simulink model "PubIfDecisionLM_MDL"  (R2020b)
settings: configuration reference "DspaceConfig" (kept outside this file)
PostLoadFcn:
  | if any(exist('dsrtsu_mdlpostloadfcn', 'file') ~= 0), dsrtsu_mdlpostloadfcn('Execute', bdroot); end
InitFcn:
  | , if any(exist('dsmpb_private', 'file') ~= 0), dsmpb_private('dsmpb_mdlclblib', 'Init', bdroot); end,
undefined symbols (not defined in the file or in its folder): OFM_OBJ_FUSIONTYPE_E, OFM_OBJ_MOVINGSTATE_E, OFM_OBJ_ORIENTATION_E, OFM_OBJ_TYPE_E, P_LM_Cyc, P_LM_EMLHistKapRcdBufSize, P_LM_EMLHistTrajBaseDis, P_LM_EMLHistTrajPNum, P_LM_EMLKapCorrMaxThre, P_LM_EMLMinKapThre, P_LM_EMLPathDisDiffThre, P_LM_EMLQuaFiltPar, P_LM_EMLTurnActKapThre, P_LM_EMLValidQuaThre, P_LM_FntPath1Disgap, P_LM_FntPath1MinDis, P_LM_FntPath1Timegap, P_LM_FntPath2Disgap, P_LM_FntPath2MinDis, P_LM_FntPath2Timegap, P_LM_FntPath3Disgap, P_LM_FntPath3MinDis, P_LM_FntPath3Timegap, P_LM_FusBLParFiltP, P_LM_FusEVDifC2Thre, P_LM_FusEVOPath1AllVSLDisThre, P_LM_FusEVOPath1AllVSLLostNumThre, P_LM_FusEVOPath1AllVSLQuaThre, P_LM_FusEVOPath1OTLFacNLC, P_LM_FusOTLQuaThre, P_LM_FusOTLSW, P_LM_FusParC0Index, P_LM_FusParC1Index, P_LM_FusParC2Index, P_LM_FusParC3Index, P_LM_FusVSLQuaThre, P_LM_FusVSLSW, P_LM_FusVSLValidSteerWheerAngThre, P_LM_FusVSLValidVxvThre, P_LM_LaneWidth, P_LM_OTLBufTPInfoEvaFactor, P_LM_OTLObjNum, P_LM_OTLObjSelectAgeThre, P_LM_OTLObjSelectDxAssessVx, P_LM_OTLObjSelectDxThre, P_LM_OTLObjSelectVxThre, P_LM_OTLObjSelectVyAssessDx, P_LM_OTLObjSelectVyThre, P_LM_OTLTrajPntBaseDis, P_LM_OTLTrajStdThre, P_LM_VSLAvailLineNum, P_LM_VSLBLSDiffThre, P_LM_VSLBLSDisRatio, P_LM_VSLFusBLParFiltP_C1, P_LM_VSLFusBLParFiltP_C2, P_LM_VSLFusBLParFiltP_C3, P_LM_VSLFusBLParFiltP_Quality, P_LM_VSLHistTrajBaseDis, P_LM_VSLHistTrajPNum, P_LM_VSLLCC0diff ... (+18)
libraries: simulink x145, LM_LIB x43
(part 12 of 24)

== system PubIfDecisionLM_MDL/Subsystem2/LM_Fusion1/LM_FusRatioCalc/LM_Fusion_EVO/LM_FusEVORatioCalc/LM_Fusion_FntPathK ==
  LM_EMLFntPath1Quality : Inport
  LM_EMLFntPath2Quality : Inport  Port=2
  LM_EMLFntPath3Quality : Inport  Port=3
  LM_VSLFntPath1Quality : Inport  Port=4
  LM_VSLFntPath2Quality : Inport  Port=5
  LM_VSLFntPath3Quality : Inport  Port=6
  LM_VSLBaseDis : Inport  Port=7
  LM_OTLFntPath1Qulity : Inport  Port=8
  LM_OTLFntPath2Qulity : Inport  Port=9
  LM_OTLFntPath3Qulity : Inport  Port=10
  LM_ComLineLostNum : Inport  Port=11
  LM_FntPath1Dis : Inport  Port=12
  LM_FntPath2Dis : Inport  Port=13
  vxvRefMs : Inport  Port=14
  DIR_TurnLeftValid : Inport  Port=15
  DIR_TurnRightValid : Inport  Port=16
  DIR_LC2LeValid : Inport  Port=17
  DIR_LC2RigValid : Inport  Port=18
  LM_FusEVOFntPath1 : Subsystem
  LM_FusEVOFntPath2 : Subsystem
  LM_FusEVOFntPath3 : Subsystem
  LM_FusEVOFntPath1EMLK : Outport
  LM_FusEVOFntPath1VSLK : Outport  Port=2
  LM_FusEVOFntPath1OTLK : Outport  Port=3
  LM_FusEVOFntPath1RELK : Outport  Port=4
  LM_FusEVOFntPath1MALK : Outport  Port=5
  LM_FusEVOFntPath2EMLK : Outport  Port=6
  LM_FusEVOFntPath2VSLK : Outport  Port=7
  LM_FusEVOFntPath2OTLK : Outport  Port=8
  LM_FusEVOFntPath2RELK : Outport  Port=9
  LM_FusEVOFntPath2MALK : Outport  Port=10
  LM_FusEVOFntPath3EMLK : Outport  Port=11
  LM_FusEVOFntPath3VSLK : Outport  Port=12
  LM_FusEVOFntPath3OTLK : Outport  Port=13
  LM_FusEVOFntPath3RELK : Outport  Port=14
  LM_FusEVOFntPath3MALK : Outport  Port=15
  wires:
  LM_EMLFntPath1Quality/1 -> LM_FusEVOFntPath1/1(LM_EMLFntPath1Quality)
  LM_VSLFntPath1Quality/1 -> LM_FusEVOFntPath1/2(LM_VSLFntPath1Quality)
  LM_VSLBaseDis/1 -> LM_FusEVOFntPath2/7(LM_VSLBaseDis), LM_FusEVOFntPath1/3(LM_VSLBaseDis)
  LM_OTLFntPath1Qulity/1 -> LM_FusEVOFntPath1/4(LM_OTLFntPath1Qulity)
  LM_ComLineLostNum/1 -> LM_FusEVOFntPath3/1(LM_ComLineLostNum), LM_FusEVOFntPath2/1(LM_ComLineLostNum), LM_FusEVOFntPath1/5(LM_ComLineLostNum)
  LM_FntPath1Dis/1 -> LM_FusEVOFntPath1/6(LM_FntPath1Dis)
  vxvRefMs/1 -> LM_FusEVOFntPath3/7(vxvRefMs), LM_FusEVOFntPath2/9(vxvRefMs), LM_FusEVOFntPath1/7(vxvRefMs)
  LM_EMLFntPath2Quality/1 -> LM_FusEVOFntPath2/2(LM_EMLFntPath2Quality)
  LM_VSLFntPath2Quality/1 -> LM_FusEVOFntPath2/3(LM_VSLFntPath2Quality)
  LM_OTLFntPath2Qulity/1 -> LM_FusEVOFntPath2/4(LM_OTLFntPath2Qulity)
  LM_FusEVOFntPath1/1(LM_FusEVOFntPath1EMLK) -> LM_FusEVOFntPath1EMLK/1
  LM_FusEVOFntPath1/2(LM_FusEVOFntPath1VSLK) -> LM_FusEVOFntPath1VSLK/1
  LM_FusEVOFntPath1/3(LM_FusEVOFntPath1OTLK) -> LM_FusEVOFntPath1OTLK/1
  LM_FusEVOFntPath2/1(LM_FusEVOFntPath2EMLK) -> LM_FusEVOFntPath2EMLK/1
  LM_FusEVOFntPath2/2(LM_FusEVOFntPath2VSLK) -> LM_FusEVOFntPath2VSLK/1
  LM_FusEVOFntPath2/3(LM_FusEVOFntPath2OTLK) -> LM_FusEVOFntPath2OTLK/1
  LM_FusEVOFntPath1/4(LM_FusEVOFntPath1RELK) -> LM_FusEVOFntPath1RELK/1
  LM_FusEVOFntPath1/5(LM_FusEVOFntPath1MALK) -> LM_FusEVOFntPath1MALK/1
  LM_FusEVOFntPath2/4(LM_FusEVOFntPath2RELK) -> LM_FusEVOFntPath2RELK/1
  LM_FusEVOFntPath2/5(LM_FusEVOFntPath2MALK) -> LM_FusEVOFntPath2MALK/1
  LM_OTLFntPath3Qulity/1 -> LM_FusEVOFntPath3/4(LM_OTLFntPath3Quality)
  LM_VSLFntPath3Quality/1 -> LM_FusEVOFntPath3/3(LM_VSLFntPath3Quality)
  LM_EMLFntPath3Quality/1 -> LM_FusEVOFntPath3/2(LM_EMLFntPath3Quality)
  LM_FusEVOFntPath3/1(LM_FusEVOFntPath3EMLK) -> LM_FusEVOFntPath3EMLK/1
  LM_FusEVOFntPath3/2(LM_FusEVOFntPath3VSLK) -> LM_FusEVOFntPath3VSLK/1
  LM_FusEVOFntPath3/3(LM_FusEVOFntPath3OTLK) -> LM_FusEVOFntPath3OTLK/1
  LM_FusEVOFntPath3/4(LM_FusEVOFntPath3RELK) -> LM_FusEVOFntPath3RELK/1
  LM_FusEVOFntPath3/5(LM_FusEVOFntPath3MALK) -> LM_FusEVOFntPath3MALK/1
  DIR_TurnLeftValid/1 -> LM_FusEVOFntPath2/5(DIR_TurnLeftValid), LM_FusEVOFntPath3/5(DIR_TurnLeftValid), LM_FusEVOFntPath1/8(DIR_TurnLeftValid)
  DIR_TurnRightValid/1 -> LM_FusEVOFntPath3/6(DIR_TurnRightValid), LM_FusEVOFntPath2/6(DIR_TurnRightValid), LM_FusEVOFntPath1/9(DIR_TurnRightValid)
  DIR_LC2LeValid/1 -> LM_FusEVOFntPath1/10(DIR_LC2LeValid), LM_FusEVOFntPath2/10(DIR_LC2LeValid), LM_FusEVOFntPath3/8(DIR_LC2LeValid)
  DIR_LC2RigValid/1 -> LM_FusEVOFntPath1/11(DIR_LC2RigValid), LM_FusEVOFntPath2/11(DIR_LC2RigValid), LM_FusEVOFntPath3/9(DIR_LC2RigValid)
  LM_FntPath2Dis/1 -> LM_FusEVOFntPath2/8(LM_FntPath2Dis)

== system PubIfDecisionLM_MDL/Subsystem2/LM_Fusion1/LM_FusRatioCalc/LM_Fusion_EVO/LM_FusEVORatioCalc/LM_Fusion_RearPathK ==
  Constant{,1..5} (6 alike) : Constant  Value=0  OutDataTypeStr=single
  LM_FusRearPath1VSLK : Outport
  LM_FusRearPath2VSLK : Outport  Port=2
  LM_FusRearPath3VSLK : Outport  Port=3
  LM_FusRearPath1EMLK : Outport  Port=4
  LM_FusRearPath2EMLK : Outport  Port=5
  LM_FusRearPath3EMLK : Outport  Port=6
  wires:
  Constant3/1 -> LM_FusRearPath2EMLK/1  "LM_FusRearPath2EMLK"
  Constant4/1 -> LM_FusRearPath3VSLK/1  "LM_FusRearPath3VSLK"
  Constant5/1 -> LM_FusRearPath3EMLK/1  "LM_FusRearPath3EMLK"
  Constant2/1 -> LM_FusRearPath2VSLK/1  "LM_FusRearPath2VSLK"
  Constant1/1 -> LM_FusRearPath1EMLK/1  "LM_FusRearPath1EMLK"
  Constant/1 -> LM_FusRearPath1VSLK/1  "LM_FusRearPath1VSLK"

== system PubIfDecisionLM_MDL/Subsystem2/LM_Fusion1/LM_Fus_BLConnectivityCheck/LM_Fus_BLFntPahtConnectivityCheck/LM_Fus_BLFntPahtConnectivityCheck/LM_Fus_BLFntPath1Info ==
  LM_FusBLFntPath1Quality : Inport
  LM_FusBLFntPath1C0 : Inport  Port=2
  LM_FusBLFntPath1C1 : Inport  Port=3
  LM_FusBLFntPath1C2 : Inport  Port=4
  LM_FusBLFntPath1C3 : Inport  Port=5
  Signal Conversion{,1..4} (5 alike) : SignalConversion  OverrideOpt=off
  LM_FusBLFntPath1C0Adju : Outport
  LM_FusBLFntPath1C1Adju : Outport  Port=2
  LM_FusBLFntPath1C2Adju : Outport  Port=3
  LM_FusBLFntPath1C3Adju : Outport  Port=4
  LM_FusBLFntPath1QualityAdju : Outport  Port=5
  wires:
  LM_FusBLFntPath1C2/1 -> Signal Conversion2/1
  LM_FusBLFntPath1C0/1 -> Signal Conversion/1
  LM_FusBLFntPath1C1/1 -> Signal Conversion1/1
  LM_FusBLFntPath1Quality/1 -> Signal Conversion4/1
  LM_FusBLFntPath1C3/1 -> Signal Conversion3/1
  Signal Conversion/1 -> LM_FusBLFntPath1C0Adju/1  "LM_FusBLFntPath1C0Adju"
  Signal Conversion1/1 -> LM_FusBLFntPath1C1Adju/1  "LM_FusBLFntPath1C1Adju"
  Signal Conversion2/1 -> LM_FusBLFntPath1C2Adju/1  "LM_FusBLFntPath1C2Adju"
  Signal Conversion3/1 -> LM_FusBLFntPath1C3Adju/1  "LM_FusBLFntPath1C3Adju"
  Signal Conversion4/1 -> LM_FusBLFntPath1QualityAdju/1  "LM_FusBLFntPath1QualityAdju"

== system PubIfDecisionLM_MDL/Subsystem2/LM_Fusion1/LM_Fus_BLConnectivityCheck/LM_Fus_BLFntPahtConnectivityCheck/LM_Fus_BLFntPahtConnectivityCheck/LM_Fus_BLFntPath2Info ==
  LM_FusBLFntPath1C0 : Inport
  LM_FusBLFntPath1C1 : Inport  Port=2
  LM_FusBLFntPath1C2 : Inport  Port=3
  LM_FusBLFntPath1C3 : Inport  Port=4
  LM_FusBLFntPath2Quality : Inport  Port=5
  LM_FusBLFntPath2C0BefAduj : Inport  Port=6
  LM_FusBLFntPath2C1 : Inport  Port=7
  LM_FusBLFntPath2C2 : Inport  Port=8
  LM_FusBLFntPath2C3 : Inport  Port=9
  LM_FntPath1Dis : Inport  Port=10
  LM_Fus_BLFntPath2C0Adju : Subsystem
  LM_Fus_BLFntPath2Info : Subsystem
  LM_FusBLFntPath2C0Adju : Outport
  LM_FusBLFntPath2C1Adju : Outport  Port=2
  LM_FusBLFntPath2C2Adju : Outport  Port=3
  LM_FusBLFntPath2C3Adju : Outport  Port=4
  LM_FusBLFntPath2QualityAdju : Outport  Port=5
  wires:
  LM_FusBLFntPath1C0/1 -> LM_Fus_BLFntPath2C0Adju/1(LM_FusBLFntPath1C0)
  LM_FusBLFntPath1C1/1 -> LM_Fus_BLFntPath2C0Adju/2(LM_FusBLFntPath1C1)
  LM_FusBLFntPath1C2/1 -> LM_Fus_BLFntPath2C0Adju/3(LM_FusBLFntPath1C2)
  LM_FusBLFntPath1C3/1 -> LM_Fus_BLFntPath2C0Adju/4(LM_FusBLFntPath1C3)
  LM_FntPath1Dis/1 -> LM_Fus_BLFntPath2C0Adju/5(LM_FntPath1Dis)
  LM_FusBLFntPath2C0BefAduj/1 -> LM_Fus_BLFntPath2C0Adju/6(LM_FusBLFntPath2C0BefAduj)
  LM_FusBLFntPath2C1/1 -> LM_Fus_BLFntPath2C0Adju/7(LM_FusBLFntPath2C1), LM_Fus_BLFntPath2Info/2(LM_FusBLFntPath2C1)
  LM_FusBLFntPath2C2/1 -> LM_Fus_BLFntPath2C0Adju/8(LM_FusBLFntPath2C2), LM_Fus_BLFntPath2Info/3(LM_FusBLFntPath2C2)
  LM_FusBLFntPath2C3/1 -> LM_Fus_BLFntPath2C0Adju/9(LM_FusBLFntPath2C3), LM_Fus_BLFntPath2Info/4(LM_FusBLFntPath2C3)
  LM_Fus_BLFntPath2C0Adju/1(LM_FusBLFntPath2C0Aduj) -> LM_Fus_BLFntPath2Info/1(LM_FusBLFntPath2C0Aduj)
  LM_FusBLFntPath2Quality/1 -> LM_Fus_BLFntPath2Info/5(LM_FusBLFntPath2Quality)
  LM_Fus_BLFntPath2Info/5(LM_FusBLFntPath2QualityAdju) -> LM_FusBLFntPath2QualityAdju/1
  LM_Fus_BLFntPath2Info/4(LM_FusBLFntPath2C3Adju) -> LM_FusBLFntPath2C3Adju/1
  LM_Fus_BLFntPath2Info/2(LM_FusBLFntPath2C1Adju) -> LM_FusBLFntPath2C1Adju/1
  LM_Fus_BLFntPath2Info/3(LM_FusBLFntPath2C2Adju) -> LM_FusBLFntPath2C2Adju/1
  LM_Fus_BLFntPath2Info/1(LM_FusBLFntPath2C0Adju) -> LM_FusBLFntPath2C0Adju/1

== system PubIfDecisionLM_MDL/Subsystem2/LM_Fusion1/LM_Fus_BLConnectivityCheck/LM_Fus_BLFntPahtConnectivityCheck/LM_Fus_BLFntPahtConnectivityCheck/LM_Fus_BLFntPath3Info ==
  LM_FusBLFntPath2C0Aduj : Inport
  LM_FusBLFntPath2C1 : Inport  Port=2
  LM_FusBLFntPath2C2 : Inport  Port=3
  LM_FusBLFntPath2C3 : Inport  Port=4
  LM_FusBLFntPath3C0BefAduj : Inport  Port=5
  LM_FusBLFntPath3C1 : Inport  Port=6
  LM_FusBLFntPath3C2 : Inport  Port=7
  LM_FusBLFntPath3C3 : Inport  Port=8
  LM_FusBLFntPath3Quality : Inport  Port=9
  LM_FntPath2Dis : Inport  Port=10
  LM_Fus_BLFntPath2C0Adju : Subsystem
  LM_Fus_BLFntPath2Info : Subsystem
  LM_FusBLFntPath3C0Adju : Outport
  LM_FusBLFntPath3C1Adju : Outport  Port=2
  LM_FusBLFntPath3C2Adju : Outport  Port=3
  LM_FusBLFntPath3C3Adju : Outport  Port=4
  LM_FusBLFntPath3QualityAdju : Outport  Port=5
  wires:
  LM_Fus_BLFntPath2C0Adju/1(LM_FusBLFntPath3C0Aduj) -> LM_Fus_BLFntPath2Info/1(LM_FusBLFntPath3C0Aduj)
  LM_FusBLFntPath3Quality/1 -> LM_Fus_BLFntPath2Info/5(LM_FusBLFntPath3Quality)
  LM_FusBLFntPath3C1/1 -> LM_Fus_BLFntPath2Info/2(LM_FusBLFntPath3C1), LM_Fus_BLFntPath2C0Adju/7(LM_FusBLFntPath3C1)
  LM_FusBLFntPath3C2/1 -> LM_Fus_BLFntPath2Info/3(LM_FusBLFntPath3C2), LM_Fus_BLFntPath2C0Adju/8(LM_FusBLFntPath3C2)
  LM_FusBLFntPath3C3/1 -> LM_Fus_BLFntPath2Info/4(LM_FusBLFntPath3C3), LM_Fus_BLFntPath2C0Adju/9(LM_FusBLFntPath3C3)
  LM_FusBLFntPath2C0Aduj/1 -> LM_Fus_BLFntPath2C0Adju/1(LM_FusBLFntPath2C0)
  LM_FusBLFntPath2C1/1 -> LM_Fus_BLFntPath2C0Adju/2(LM_FusBLFntPath2C1)
  LM_FusBLFntPath2C2/1 -> LM_Fus_BLFntPath2C0Adju/3(LM_FusBLFntPath2C2)
  LM_FusBLFntPath2C3/1 -> LM_Fus_BLFntPath2C0Adju/4(LM_FusBLFntPath2C3)
  LM_FntPath2Dis/1 -> LM_Fus_BLFntPath2C0Adju/5(LM_FntPath2Dis)
  LM_FusBLFntPath3C0BefAduj/1 -> LM_Fus_BLFntPath2C0Adju/6(LM_FusBLFntPath3C0BefAduj)
  LM_Fus_BLFntPath2Info/3(LM_FusBLFntPath3C2Adju) -> LM_FusBLFntPath3C2Adju/1
  LM_Fus_BLFntPath2Info/2(LM_FusBLFntPath3C1Adju) -> LM_FusBLFntPath3C1Adju/1
  LM_Fus_BLFntPath2Info/4(LM_FusBLFntPath3C3Adju) -> LM_FusBLFntPath3C3Adju/1
  LM_Fus_BLFntPath2Info/1(LM_FusBLFntPath3C0Adju) -> LM_FusBLFntPath3C0Adju/1
  LM_Fus_BLFntPath2Info/5(LM_FusBLFntPath3QualityAdju) -> LM_FusBLFntPath3QualityAdju/1

== system PubIfDecisionLM_MDL/Subsystem2/LM_Fusion1/LM_Fus_BLConnectivityCheck/LM_Fus_BLRearPahtConnectivityCheck/LM_Fus_BLRearPahtConnectivityCheck/LM_Fus_BLFntPath2Info ==
  LM_FusBLRearPath1C0 : Inport
  LM_FusBLRearPath1C1 : Inport  Port=2
  LM_FusBLRearPath1C2 : Inport  Port=3
  LM_FusBLRearPath1C3 : Inport  Port=4
  LM_FusBLRearPath2Quality : Inport  Port=5
  LM_FusBLFntPath2C0BefAduj : Inport  Port=6
  LM_FusBLRearPath2C1 : Inport  Port=7
  LM_FusBLRearPath2C2 : Inport  Port=8
  LM_FusBLRearPath2C3 : Inport  Port=9
  LM_RearPath1Dis : Inport  Port=10
  LM_Fus_BLFntPath2C0Adju : Subsystem
  LM_Fus_BLFntPath2Info : Subsystem
  LM_FusBLRearPath2C0Adju : Outport
  LM_FusBLRearPath2C1Adju : Outport  Port=2
  LM_FusBLRearPath2C2Adju : Outport  Port=3
  LM_FusBLRearPath2C3Adju : Outport  Port=4
  LM_FusBLRearPath2QualityAdju : Outport  Port=5
  wires:
  LM_FusBLRearPath1C0/1 -> LM_Fus_BLFntPath2C0Adju/1(LM_FusBLFntPath1C0)
  LM_FusBLRearPath1C1/1 -> LM_Fus_BLFntPath2C0Adju/2(LM_FusBLFntPath1C1)
  LM_FusBLRearPath1C2/1 -> LM_Fus_BLFntPath2C0Adju/3(LM_FusBLFntPath1C2)
  LM_FusBLRearPath1C3/1 -> LM_Fus_BLFntPath2C0Adju/4(LM_FusBLFntPath1C3)
  LM_RearPath1Dis/1 -> LM_Fus_BLFntPath2C0Adju/5(LM_FntPath1Dis)
  LM_FusBLFntPath2C0BefAduj/1 -> LM_Fus_BLFntPath2C0Adju/6(LM_FusBLFntPath2C0BefAduj)
  LM_FusBLRearPath2C1/1 -> LM_Fus_BLFntPath2C0Adju/7(LM_FusBLFntPath2C1), LM_Fus_BLFntPath2Info/2(LM_FusBLFntPath2C1)
  LM_FusBLRearPath2C2/1 -> LM_Fus_BLFntPath2C0Adju/8(LM_FusBLFntPath2C2), LM_Fus_BLFntPath2Info/3(LM_FusBLFntPath2C2)
  LM_FusBLRearPath2C3/1 -> LM_Fus_BLFntPath2C0Adju/9(LM_FusBLFntPath2C3), LM_Fus_BLFntPath2Info/4(LM_FusBLFntPath2C3)
  LM_Fus_BLFntPath2C0Adju/1(LM_FusBLFntPath2C0Aduj) -> LM_Fus_BLFntPath2Info/1(LM_FusBLFntPath2C0Aduj)
  LM_FusBLRearPath2Quality/1 -> LM_Fus_BLFntPath2Info/5(LM_FusBLFntPath2Quality)
  LM_Fus_BLFntPath2Info/5(LM_FusBLRearPath2QualityAdju) -> LM_FusBLRearPath2QualityAdju/1
  LM_Fus_BLFntPath2Info/4(LM_FusBLRearPath2C3Adju) -> LM_FusBLRearPath2C3Adju/1
  LM_Fus_BLFntPath2Info/2(LM_FusBLRearPath2C1Adju) -> LM_FusBLRearPath2C1Adju/1
  LM_Fus_BLFntPath2Info/3(LM_FusBLRearPath2C2Adju) -> LM_FusBLRearPath2C2Adju/1
  LM_Fus_BLFntPath2Info/1(LM_FusBLRearPath2C0Adju) -> LM_FusBLRearPath2C0Adju/1

== system PubIfDecisionLM_MDL/Subsystem2/LM_Fusion1/LM_Fus_BLConnectivityCheck/LM_Fus_BLRearPahtConnectivityCheck/LM_Fus_BLRearPahtConnectivityCheck/LM_Fus_BLFntPath3Info ==
  LM_FusBLFntPath2C0Aduj : Inport
  LM_FusBLFntPath2C1 : Inport  Port=2
  LM_FusBLFntPath2C2 : Inport  Port=3
  LM_FusBLFntPath2C3 : Inport  Port=4
  LM_FusBLFntPath3C0BefAduj : Inport  Port=5
  LM_FusBLFntPath3C1 : Inport  Port=6
  LM_FusBLFntPath3C2 : Inport  Port=7
  LM_FusBLFntPath3C3 : Inport  Port=8
  LM_FusBLFntPath3Quality : Inport  Port=9
  LM_FntPath2Dis : Inport  Port=10
  LM_Fus_BLFntPath2Info : Subsystem
  LM_Fus_BLRearPath3C0Adju : Subsystem
  LM_FusBLRearPath3C0Adju : Outport
  LM_FusBLRearPath3C1Adju : Outport  Port=2
  LM_FusBLRearPath3C2Adju : Outport  Port=3
  LM_FusBLRearPath3C3Adju : Outport  Port=4
  LM_FusBLRearPath3QualityAdju : Outport  Port=5
  wires:
  LM_Fus_BLRearPath3C0Adju/1(LM_FusBLFntPath3C0Check) -> LM_Fus_BLFntPath2Info/1(LM_FusBLFntPath3C0Check)
  LM_FusBLFntPath3Quality/1 -> LM_Fus_BLFntPath2Info/5(LM_FusBLFntPath3Quality)
  LM_FusBLFntPath3C1/1 -> LM_Fus_BLFntPath2Info/2(LM_FusBLFntPath3C1), LM_Fus_BLRearPath3C0Adju/7(LM_FusBLFntPath3C1)
  LM_FusBLFntPath3C2/1 -> LM_Fus_BLFntPath2Info/3(LM_FusBLFntPath3C2), LM_Fus_BLRearPath3C0Adju/8(LM_FusBLFntPath3C2)
  LM_FusBLFntPath3C3/1 -> LM_Fus_BLFntPath2Info/4(LM_FusBLFntPath3C3), LM_Fus_BLRearPath3C0Adju/9(LM_FusBLFntPath3C3)
  LM_FusBLFntPath2C0Aduj/1 -> LM_Fus_BLRearPath3C0Adju/1(LM_FusBLFntPath2C0)
  LM_FusBLFntPath2C1/1 -> LM_Fus_BLRearPath3C0Adju/2(LM_FusBLFntPath2C1)
  LM_FusBLFntPath2C2/1 -> LM_Fus_BLRearPath3C0Adju/3(LM_FusBLFntPath2C2)
  LM_FusBLFntPath2C3/1 -> LM_Fus_BLRearPath3C0Adju/4(LM_FusBLFntPath2C3)
  LM_FntPath2Dis/1 -> LM_Fus_BLRearPath3C0Adju/5(LM_FntPath2Dis)
  LM_FusBLFntPath3C0BefAduj/1 -> LM_Fus_BLRearPath3C0Adju/6(LM_FusBLFntPath3C0BefAduj)
  LM_Fus_BLFntPath2Info/2(LM_FusBLRearPath3C1Adju) -> LM_FusBLRearPath3C1Adju/1
  LM_Fus_BLFntPath2Info/3(LM_FusBLRearPath3C2Adju) -> LM_FusBLRearPath3C2Adju/1
  LM_Fus_BLFntPath2Info/1(LM_FusBLRearPath3C0Adju) -> LM_FusBLRearPath3C0Adju/1
  LM_Fus_BLFntPath2Info/4(LM_FusBLRearPath3C3Adju) -> LM_FusBLRearPath3C3Adju/1
  LM_Fus_BLFntPath2Info/5(LM_FusBLRearPath3QualityAdju) -> LM_FusBLRearPath3QualityAdju/1

== system PubIfDecisionLM_MDL/Subsystem2/LM_Fusion1/LM_Fus_BLConnectivityCheck/LM_Fus_BLRearPahtConnectivityCheck/LM_Fus_BLRearPahtConnectivityCheck/LM_Fus_BLRearPath1Info ==
  LM_FusBLFntPath1Quality : Inport
  LM_FusBLFntPath1C0 : Inport  Port=2
  LM_FusBLFntPath1C1 : Inport  Port=3
  LM_FusBLFntPath1C2 : Inport  Port=4
  LM_FusBLFntPath1C3 : Inport  Port=5
  Signal Conversion{,1..4} (5 alike) : SignalConversion  OverrideOpt=off
  LM_FusBLRearPath1C0Adju : Outport
  LM_FusBLRearPath1C1Adju : Outport  Port=2
  LM_FusBLRearPath1C2Adju : Outport  Port=3
  LM_FusBLRearPath1C3Adju : Outport  Port=4
  LM_FusBLRearPath1QualityAdju : Outport  Port=5
  wires:
  Signal Conversion/1 -> LM_FusBLRearPath1C0Adju/1  "LM_FusBLRearPath1C0Adju"
  Signal Conversion2/1 -> LM_FusBLRearPath1C2Adju/1  "LM_FusBLRearPath1C2Adju"
  Signal Conversion4/1 -> LM_FusBLRearPath1QualityAdju/1  "LM_FusBLRearPath1QualityAdju"
  Signal Conversion3/1 -> LM_FusBLRearPath1C3Adju/1  "LM_FusBLRearPath1C3Adju"
  Signal Conversion1/1 -> LM_FusBLRearPath1C1Adju/1  "LM_FusBLRearPath1C1Adju"
  LM_FusBLFntPath1C0/1 -> Signal Conversion/1
  LM_FusBLFntPath1C1/1 -> Signal Conversion1/1
  LM_FusBLFntPath1C2/1 -> Signal Conversion2/1
  LM_FusBLFntPath1C3/1 -> Signal Conversion3/1
  LM_FusBLFntPath1Quality/1 -> Signal Conversion4/1

== system PubIfDecisionLM_MDL/Subsystem2/LM_OTL/LM_OTL_MovObjTrajFit/LM_OTL_BufTPAssess/LM_OTL_BufTrajEva/Subsystem ==
  LM_OTLBufValid : Inport
  LM_OTLBufTPVectBus : Inport  Port=2
  ILM_OTLBufTPInfoBus : Inport  Port=3
  LM_PathDisBus : Inport  Port=4
  Bus Selector : BusSelector  OutputSignals=LM_OTLBufE1Valid
  Bus Selector1 : BusSelector  OutputSignals=LM_OTLBufE1DxVect,LM_OTLBufE1DyVect
  Bus Selector2 : BusSelector  OutputSignals=LM_OTLBufSPPosInfo.LM_OTLBufE1SPPos,LM_OTLBufEPPosInfo.LM_OTLBufE1EPPos
  Bus Selector3 : BusSelector  OutputSignals=LM_PathDisBus.LM_FntPath1Dis,LM_PathDisBus.LM_FntPath2Dis,LM_PathDisBus.LM_FntPath3Dis
  Constant : Constant  Value=P_LM_OTLTrajStdThre
  MATLAB Function1 : MATLAB Function  TreatAsAtomicUnit=on
  LM_OTLBufE1Offset : Outport
  LM_OTLBufE1Flg : Outport  Port=2
  LM_OTLBufE1TpValidNum : Outport  Port=3
  LM_OTLBufE1SPValidPos : Outport  Port=4
  wires:
  Constant/1 -> MATLAB Function1/9(P_LM_OTLTrajStdThre)
  Bus Selector1/1 -> MATLAB Function1/2(LM_OTLDxVect)  "<LM_OTLBufE1DxVect>"
  Bus Selector/1 -> MATLAB Function1/1(LM_OTLBufValidInfo)  "<LM_OTLBufE1Valid>"
  MATLAB Function1/2(Flg) -> LM_OTLBufE1Flg/1
  Bus Selector3/3 -> MATLAB Function1/8(LM_FntPath3Dis)  "<LM_FntPath3Dis>"
  Bus Selector2/1 -> MATLAB Function1/4(LM_OTLSPPos)  "<LM_OTLBufE1SPPos>"
  Bus Selector2/2 -> MATLAB Function1/5(LM_OTLEPPos)  "<LM_OTLBufE1EPPos>"
  Bus Selector1/2 -> MATLAB Function1/3(LM_OTLDyVect)  "<LM_OTLBufE1DyVect>"
  LM_OTLBufValid/1 -> Bus Selector/1
  Bus Selector3/2 -> MATLAB Function1/7(LM_FntPath2Dis)  "<LM_FntPath2Dis>"
  Bus Selector3/1 -> MATLAB Function1/6(LM_FntPath1Dis)  "<LM_FntPath1Dis>"
  MATLAB Function1/1(Offset) -> LM_OTLBufE1Offset/1
  ILM_OTLBufTPInfoBus/1 -> Bus Selector2/1
  LM_OTLBufTPVectBus/1 -> Bus Selector1/1
  LM_PathDisBus/1 -> Bus Selector3/1
  MATLAB Function1/3(TpValidNum) -> LM_OTLBufE1TpValidNum/1
  MATLAB Function1/4(SPValidPos) -> LM_OTLBufE1SPValidPos/1

== system PubIfDecisionLM_MDL/Subsystem2/LM_OTL/LM_OTL_MovObjTrajFit/LM_OTL_BufTPAssess/LM_OTL_BufTrajEva/Subsystem1 ==
  LM_OTLBufValid : Inport
  LM_OTLBufTPVectBus : Inport  Port=2
  ILM_OTLBufTPInfoBus : Inport  Port=3
  LM_PathDisBus : Inport  Port=4
  Bus Selector : BusSelector  OutputSignals=LM_OTLBufL1LastValid
  Bus Selector1 : BusSelector  OutputSignals=LM_OTLBufL1DxVect,LM_OTLBufL1DyVect
  Bus Selector2 : BusSelector  OutputSignals=LM_OTLBufLastSPPosInfo.LM_OTLBufL1LastSPPos,LM_OTLBufLastEPPosInfo.LM_OTLBufL1LastEPPos
  Bus Selector3 : BusSelector  OutputSignals=LM_PathDisBus.LM_FntPath1Dis,LM_PathDisBus.LM_FntPath2Dis,LM_PathDisBus.LM_FntPath3Dis
  Constant : Constant  Value=P_LM_OTLTrajStdThre
  MATLAB Function1 : MATLAB Function  TreatAsAtomicUnit=on
  LM_OTLBufL1LastOffset : Outport
  LM_OTLBufL1LastFlg : Outport  Port=2
  LM_OTLBufL1TpLastValidNum : Outport  Port=3
  LM_OTLBufL1SPLastValidPos : Outport  Port=4
  wires:
  Constant/1 -> MATLAB Function1/9(P_LM_OTLTrajStdThre)
  Bus Selector1/1 -> MATLAB Function1/2(LM_OTLDxVect)  "<LM_OTLBufL1DxVect>"
  Bus Selector/1 -> MATLAB Function1/1(LM_OTLBufValidInfo)  "<LM_OTLBufL1LastValid>"
  MATLAB Function1/2(Flg) -> LM_OTLBufL1LastFlg/1
  Bus Selector3/3 -> MATLAB Function1/8(LM_FntPath3Dis)  "<LM_FntPath3Dis>"
  Bus Selector2/1 -> MATLAB Function1/4(LM_OTLSPPos)  "<LM_OTLBufL1LastSPPos>"
  Bus Selector2/2 -> MATLAB Function1/5(LM_OTLEPPos)  "<LM_OTLBufL1LastEPPos>"
  Bus Selector1/2 -> MATLAB Function1/3(LM_OTLDyVect)  "<LM_OTLBufL1DyVect>"
  LM_OTLBufValid/1 -> Bus Selector/1
  Bus Selector3/2 -> MATLAB Function1/7(LM_FntPath2Dis)  "<LM_FntPath2Dis>"
  Bus Selector3/1 -> MATLAB Function1/6(LM_FntPath1Dis)  "<LM_FntPath1Dis>"
  MATLAB Function1/1(Offset) -> LM_OTLBufL1LastOffset/1
  ILM_OTLBufTPInfoBus/1 -> Bus Selector2/1
  LM_OTLBufTPVectBus/1 -> Bus Selector1/1
  LM_PathDisBus/1 -> Bus Selector3/1
  MATLAB Function1/4(SPValidPos) -> LM_OTLBufL1SPLastValidPos/1
  MATLAB Function1/3(TpValidNum) -> LM_OTLBufL1TpLastValidNum/1

== system PubIfDecisionLM_MDL/Subsystem2/LM_OTL/LM_OTL_MovObjTrajFit/LM_OTL_BufTPAssess/LM_OTL_BufTrajEva/Subsystem10 ==
  LM_OTLBufValid : Inport
  LM_OTLBufTPVectBus : Inport  Port=2
  ILM_OTLBufTPInfoBus : Inport  Port=3
  LM_PathDisBus : Inport  Port=4
  Bus Selector : BusSelector  OutputSignals=LM_OTLBufR2LastValid
  Bus Selector1 : BusSelector  OutputSignals=LM_OTLBufR2DxVect,LM_OTLBufR2DyVect
  Bus Selector2 : BusSelector  OutputSignals=LM_OTLBufLastSPPosInfo.LM_OTLBufR2LastSPPos,LM_OTLBufLastEPPosInfo.LM_OTLBufR2LastEPPos
  Bus Selector3 : BusSelector  OutputSignals=LM_PathDisBus.LM_FntPath1Dis,LM_PathDisBus.LM_FntPath2Dis,LM_PathDisBus.LM_FntPath3Dis
  Constant : Constant  Value=P_LM_OTLTrajStdThre
  MATLAB Function1 : MATLAB Function  TreatAsAtomicUnit=on
  LM_OTLBufR2LastOffset : Outport
  LM_OTLBufR2LastFlg : Outport  Port=2
  LM_OTLBufR2TpLastValidNum : Outport  Port=3
  LM_OTLBufR2SPLastValidPos : Outport  Port=4
  wires:
  Constant/1 -> MATLAB Function1/9(P_LM_OTLTrajStdThre)
  Bus Selector1/1 -> MATLAB Function1/2(LM_OTLDxVect)  "<LM_OTLBufR2DxVect>"
  Bus Selector/1 -> MATLAB Function1/1(LM_OTLBufValidInfo)  "<LM_OTLBufR2LastValid>"
  MATLAB Function1/2(Flg) -> LM_OTLBufR2LastFlg/1
  Bus Selector3/3 -> MATLAB Function1/8(LM_FntPath3Dis)  "<LM_FntPath3Dis>"
  Bus Selector2/1 -> MATLAB Function1/4(LM_OTLSPPos)  "<LM_OTLBufR2LastSPPos>"
  Bus Selector2/2 -> MATLAB Function1/5(LM_OTLEPPos)  "<LM_OTLBufR2LastEPPos>"
  Bus Selector1/2 -> MATLAB Function1/3(LM_OTLDyVect)  "<LM_OTLBufR2DyVect>"
  LM_OTLBufValid/1 -> Bus Selector/1
  Bus Selector3/2 -> MATLAB Function1/7(LM_FntPath2Dis)  "<LM_FntPath2Dis>"
  Bus Selector3/1 -> MATLAB Function1/6(LM_FntPath1Dis)  "<LM_FntPath1Dis>"
  MATLAB Function1/1(Offset) -> LM_OTLBufR2LastOffset/1
  ILM_OTLBufTPInfoBus/1 -> Bus Selector2/1
  LM_OTLBufTPVectBus/1 -> Bus Selector1/1
  LM_PathDisBus/1 -> Bus Selector3/1
  MATLAB Function1/3(TpValidNum) -> LM_OTLBufR2TpLastValidNum/1
  MATLAB Function1/4(SPValidPos) -> LM_OTLBufR2SPLastValidPos/1

== system PubIfDecisionLM_MDL/Subsystem2/LM_OTL/LM_OTL_MovObjTrajFit/LM_OTL_BufTPAssess/LM_OTL_BufTrajEva/Subsystem11 ==
  LM_OTLBufValid : Inport
  LM_OTLBufTPVectBus : Inport  Port=2
  ILM_OTLBufTPInfoBus : Inport  Port=3
  LM_PathDisBus : Inport  Port=4
  Bus Selector : BusSelector  OutputSignals=LM_OTLBufR2Valid
  Bus Selector1 : BusSelector  OutputSignals=LM_OTLBufR2DxVect,LM_OTLBufR2DyVect
  Bus Selector2 : BusSelector  OutputSignals=LM_OTLBufSPPosInfo.LM_OTLBufR2SPPos,LM_OTLBufEPPosInfo.LM_OTLBufR2EPPos
  Bus Selector3 : BusSelector  OutputSignals=LM_PathDisBus.LM_FntPath1Dis,LM_PathDisBus.LM_FntPath2Dis,LM_PathDisBus.LM_FntPath3Dis
  Constant : Constant  Value=P_LM_OTLTrajStdThre
  MATLAB Function1 : MATLAB Function  TreatAsAtomicUnit=on
  LM_OTLBufR2Offset : Outport
  LM_OTLBufR2Flg : Outport  Port=2
  LM_OTLBufR2TpValidNum : Outport  Port=3
  LM_OTLBufR2SPValidPos : Outport  Port=4
  wires:
  Constant/1 -> MATLAB Function1/9(P_LM_OTLTrajStdThre)
  Bus Selector1/1 -> MATLAB Function1/2(LM_OTLDxVect)  "<LM_OTLBufR2DxVect>"
  Bus Selector/1 -> MATLAB Function1/1(LM_OTLBufValidInfo)  "<LM_OTLBufR2Valid>"
  MATLAB Function1/2(Flg) -> LM_OTLBufR2Flg/1
  Bus Selector3/3 -> MATLAB Function1/8(LM_FntPath3Dis)  "<LM_FntPath3Dis>"
  Bus Selector2/1 -> MATLAB Function1/4(LM_OTLSPPos)  "<LM_OTLBufR2SPPos>"
  Bus Selector2/2 -> MATLAB Function1/5(LM_OTLEPPos)  "<LM_OTLBufR2EPPos>"
  Bus Selector1/2 -> MATLAB Function1/3(LM_OTLDyVect)  "<LM_OTLBufR2DyVect>"
  LM_OTLBufValid/1 -> Bus Selector/1
  Bus Selector3/2 -> MATLAB Function1/7(LM_FntPath2Dis)  "<LM_FntPath2Dis>"
  Bus Selector3/1 -> MATLAB Function1/6(LM_FntPath1Dis)  "<LM_FntPath1Dis>"
  MATLAB Function1/1(Offset) -> LM_OTLBufR2Offset/1
  ILM_OTLBufTPInfoBus/1 -> Bus Selector2/1
  LM_OTLBufTPVectBus/1 -> Bus Selector1/1
  LM_PathDisBus/1 -> Bus Selector3/1
  MATLAB Function1/3(TpValidNum) -> LM_OTLBufR2TpValidNum/1
  MATLAB Function1/4(SPValidPos) -> LM_OTLBufR2SPValidPos/1

== system PubIfDecisionLM_MDL/Subsystem2/LM_OTL/LM_OTL_MovObjTrajFit/LM_OTL_BufTPAssess/LM_OTL_BufTrajEva/Subsystem2 ==
  LM_OTLBufValid : Inport
  LM_OTLBufTPVectBus : Inport  Port=2
  ILM_OTLBufTPInfoBus : Inport  Port=3
  LM_PathDisBus : Inport  Port=4
  Bus Selector : BusSelector  OutputSignals=LM_OTLBufL1Valid
  Bus Selector1 : BusSelector  OutputSignals=LM_OTLBufL1DxVect,LM_OTLBufL1DyVect
  Bus Selector2 : BusSelector  OutputSignals=LM_OTLBufSPPosInfo.LM_OTLBufL1SPPos,LM_OTLBufEPPosInfo.LM_OTLBufL1EPPos
  Bus Selector3 : BusSelector  OutputSignals=LM_PathDisBus.LM_FntPath1Dis,LM_PathDisBus.LM_FntPath2Dis,LM_PathDisBus.LM_FntPath3Dis
  Constant : Constant  Value=P_LM_OTLTrajStdThre
  MATLAB Function1 : MATLAB Function  TreatAsAtomicUnit=on
  LM_OTLBufL1Offset : Outport
  LM_OTLBufL1Flg : Outport  Port=2
  LM_OTLBufL1TpValidNum : Outport  Port=3
  LM_OTLBufL1SPValidPos : Outport  Port=4
  wires:
  Constant/1 -> MATLAB Function1/9(P_LM_OTLTrajStdThre)
  Bus Selector1/1 -> MATLAB Function1/2(LM_OTLDxVect)  "<LM_OTLBufL1DxVect>"
  Bus Selector/1 -> MATLAB Function1/1(LM_OTLBufValidInfo)  "<LM_OTLBufL1Valid>"
  MATLAB Function1/2(Flg) -> LM_OTLBufL1Flg/1
  Bus Selector3/3 -> MATLAB Function1/8(LM_FntPath3Dis)  "<LM_FntPath3Dis>"
  Bus Selector2/1 -> MATLAB Function1/4(LM_OTLSPPos)  "<LM_OTLBufL1SPPos>"
  Bus Selector2/2 -> MATLAB Function1/5(LM_OTLEPPos)  "<LM_OTLBufL1EPPos>"
  Bus Selector1/2 -> MATLAB Function1/3(LM_OTLDyVect)  "<LM_OTLBufL1DyVect>"
  LM_OTLBufValid/1 -> Bus Selector/1
  Bus Selector3/2 -> MATLAB Function1/7(LM_FntPath2Dis)  "<LM_FntPath2Dis>"
  Bus Selector3/1 -> MATLAB Function1/6(LM_FntPath1Dis)  "<LM_FntPath1Dis>"
  MATLAB Function1/1(Offset) -> LM_OTLBufL1Offset/1
  ILM_OTLBufTPInfoBus/1 -> Bus Selector2/1
  LM_OTLBufTPVectBus/1 -> Bus Selector1/1
  LM_PathDisBus/1 -> Bus Selector3/1
  MATLAB Function1/3(TpValidNum) -> LM_OTLBufL1TpValidNum/1
  MATLAB Function1/4(SPValidPos) -> LM_OTLBufL1SPValidPos/1

== system PubIfDecisionLM_MDL/Subsystem2/LM_OTL/LM_OTL_MovObjTrajFit/LM_OTL_BufTPAssess/LM_OTL_BufTrajEva/Subsystem3 ==
  LM_OTLBufValid : Inport
  LM_OTLBufTPVectBus : Inport  Port=2
  ILM_OTLBufTPInfoBus : Inport  Port=3
  LM_PathDisBus : Inport  Port=4
  Bus Selector : BusSelector  OutputSignals=LM_OTLBufL2LastValid
  Bus Selector1 : BusSelector  OutputSignals=LM_OTLBufL2DxVect,LM_OTLBufL2DyVect
  Bus Selector2 : BusSelector  OutputSignals=LM_OTLBufLastSPPosInfo.LM_OTLBufL2LastSPPos,LM_OTLBufLastEPPosInfo.LM_OTLBufL2LastEPPos
  Bus Selector3 : BusSelector  OutputSignals=LM_PathDisBus.LM_FntPath1Dis,LM_PathDisBus.LM_FntPath2Dis,LM_PathDisBus.LM_FntPath3Dis
  Constant : Constant  Value=P_LM_OTLTrajStdThre
  MATLAB Function2 : MATLAB Function  TreatAsAtomicUnit=on
  LM_OTLBufL2LastOffset : Outport
  LM_OTLBufL2LastFlg : Outport  Port=2
  LM_OTLBufL2TpLastValidNum : Outport  Port=3
  LM_OTLBufL2SPLastValidPos : Outport  Port=4
  wires:
  Constant/1 -> MATLAB Function2/9(P_LM_OTLTrajStdThre)
  Bus Selector1/1 -> MATLAB Function2/2(LM_OTLDxVect)  "<LM_OTLBufL2DxVect>"
  Bus Selector/1 -> MATLAB Function2/1(LM_OTLBufValidInfo)  "<LM_OTLBufL2LastValid>"
  MATLAB Function2/2(Flg) -> LM_OTLBufL2LastFlg/1
  Bus Selector3/3 -> MATLAB Function2/8(LM_FntPath3Dis)  "<LM_FntPath3Dis>"
  Bus Selector2/1 -> MATLAB Function2/4(LM_OTLSPPos)  "<LM_OTLBufL2LastSPPos>"
  Bus Selector2/2 -> MATLAB Function2/5(LM_OTLEPPos)  "<LM_OTLBufL2LastEPPos>"
  Bus Selector1/2 -> MATLAB Function2/3(LM_OTLDyVect)  "<LM_OTLBufL2DyVect>"
  LM_OTLBufValid/1 -> Bus Selector/1
  Bus Selector3/2 -> MATLAB Function2/7(LM_FntPath2Dis)  "<LM_FntPath2Dis>"
  Bus Selector3/1 -> MATLAB Function2/6(LM_FntPath1Dis)  "<LM_FntPath1Dis>"
  MATLAB Function2/1(Offset) -> LM_OTLBufL2LastOffset/1
  ILM_OTLBufTPInfoBus/1 -> Bus Selector2/1
  LM_OTLBufTPVectBus/1 -> Bus Selector1/1
  LM_PathDisBus/1 -> Bus Selector3/1
  MATLAB Function2/3(TpValidNum) -> LM_OTLBufL2TpLastValidNum/1
  MATLAB Function2/4(SPValidPos) -> LM_OTLBufL2SPLastValidPos/1

== system PubIfDecisionLM_MDL/Subsystem2/LM_OTL/LM_OTL_MovObjTrajFit/LM_OTL_BufTPAssess/LM_OTL_BufTrajEva/Subsystem4 ==
  LM_OTLBufValid : Inport
  LM_OTLBufTPVectBus : Inport  Port=2
  ILM_OTLBufTPInfoBus : Inport  Port=3
  LM_PathDisBus : Inport  Port=4
  Bus Selector : BusSelector  OutputSignals=LM_OTLBufL2Valid
  Bus Selector1 : BusSelector  OutputSignals=LM_OTLBufL2DxVect,LM_OTLBufL2DyVect
  Bus Selector2 : BusSelector  OutputSignals=LM_OTLBufSPPosInfo.LM_OTLBufL2SPPos,LM_OTLBufEPPosInfo.LM_OTLBufL2EPPos
  Bus Selector3 : BusSelector  OutputSignals=LM_PathDisBus.LM_FntPath1Dis,LM_PathDisBus.LM_FntPath2Dis,LM_PathDisBus.LM_FntPath3Dis
  Constant : Constant  Value=P_LM_OTLTrajStdThre
  MATLAB Function1 : MATLAB Function  TreatAsAtomicUnit=on
  LM_OTLBufL2Offset : Outport
  LM_OTLBufL2Flg : Outport  Port=2
  LM_OTLBufL2TpValidNum : Outport  Port=3
  LM_OTLBufL2SPValidPos : Outport  Port=4
  wires:
  Constant/1 -> MATLAB Function1/9(P_LM_OTLTrajStdThre)
  Bus Selector1/1 -> MATLAB Function1/2(LM_OTLDxVect)  "<LM_OTLBufL2DxVect>"
  Bus Selector/1 -> MATLAB Function1/1(LM_OTLBufValidInfo)  "<LM_OTLBufL2Valid>"
  MATLAB Function1/2(Flg) -> LM_OTLBufL2Flg/1
  Bus Selector3/3 -> MATLAB Function1/8(LM_FntPath3Dis)  "<LM_FntPath3Dis>"
  Bus Selector2/1 -> MATLAB Function1/4(LM_OTLSPPos)  "<LM_OTLBufL2SPPos>"
  Bus Selector2/2 -> MATLAB Function1/5(LM_OTLEPPos)  "<LM_OTLBufL2EPPos>"
  Bus Selector1/2 -> MATLAB Function1/3(LM_OTLDyVect)  "<LM_OTLBufL2DyVect>"
  LM_OTLBufValid/1 -> Bus Selector/1
  Bus Selector3/2 -> MATLAB Function1/7(LM_FntPath2Dis)  "<LM_FntPath2Dis>"
  Bus Selector3/1 -> MATLAB Function1/6(LM_FntPath1Dis)  "<LM_FntPath1Dis>"
  MATLAB Function1/1(Offset) -> LM_OTLBufL2Offset/1
  ILM_OTLBufTPInfoBus/1 -> Bus Selector2/1
  LM_OTLBufTPVectBus/1 -> Bus Selector1/1
  LM_PathDisBus/1 -> Bus Selector3/1
  MATLAB Function1/3(TpValidNum) -> LM_OTLBufL2TpValidNum/1
  MATLAB Function1/4(SPValidPos) -> LM_OTLBufL2SPValidPos/1

== system PubIfDecisionLM_MDL/Subsystem2/LM_OTL/LM_OTL_MovObjTrajFit/LM_OTL_BufTPAssess/LM_OTL_BufTrajEva/Subsystem5 ==
  LM_OTLBufValid : Inport
  LM_OTLBufTPVectBus : Inport  Port=2
  ILM_OTLBufTPInfoBus : Inport  Port=3
  LM_PathDisBus : Inport  Port=4
  Bus Selector : BusSelector  OutputSignals=LM_OTLBufE1LastValid
  Bus Selector1 : BusSelector  OutputSignals=LM_OTLBufE1DxVect,LM_OTLBufE1DyVect
  Bus Selector2 : BusSelector  OutputSignals=LM_OTLBufLastSPPosInfo.LM_OTLBufE1LastSPPos,LM_OTLBufLastEPPosInfo.LM_OTLBufE1LastEPPos
  Bus Selector3 : BusSelector  OutputSignals=LM_PathDisBus.LM_FntPath1Dis,LM_PathDisBus.LM_FntPath2Dis,LM_PathDisBus.LM_FntPath3Dis
  Constant : Constant  Value=P_LM_OTLTrajStdThre
  MATLAB Function1 : MATLAB Function  TreatAsAtomicUnit=on
  LM_OTLBufE1LastOffset : Outport
  LM_OTLBufE1LastFlg : Outport  Port=2
  LM_OTLBufE1TpLastValidNum : Outport  Port=3
  LM_OTLBufE1SPLastValidPos : Outport  Port=4
  wires:
  Constant/1 -> MATLAB Function1/9(P_LM_OTLTrajStdThre)
  Bus Selector1/1 -> MATLAB Function1/2(LM_OTLDxVect)  "<LM_OTLBufE1DxVect>"
  Bus Selector/1 -> MATLAB Function1/1(LM_OTLBufValidInfo)  "<LM_OTLBufE1LastValid>"
  MATLAB Function1/2(Flg) -> LM_OTLBufE1LastFlg/1
  Bus Selector3/3 -> MATLAB Function1/8(LM_FntPath3Dis)  "<LM_FntPath3Dis>"
  Bus Selector2/1 -> MATLAB Function1/4(LM_OTLSPPos)  "<LM_OTLBufE1LastSPPos>"
  Bus Selector2/2 -> MATLAB Function1/5(LM_OTLEPPos)  "<LM_OTLBufE1LastEPPos>"
  Bus Selector1/2 -> MATLAB Function1/3(LM_OTLDyVect)  "<LM_OTLBufE1DyVect>"
  LM_OTLBufValid/1 -> Bus Selector/1
  Bus Selector3/2 -> MATLAB Function1/7(LM_FntPath2Dis)  "<LM_FntPath2Dis>"
  Bus Selector3/1 -> MATLAB Function1/6(LM_FntPath1Dis)  "<LM_FntPath1Dis>"
  MATLAB Function1/1(Offset) -> LM_OTLBufE1LastOffset/1
  ILM_OTLBufTPInfoBus/1 -> Bus Selector2/1
  LM_OTLBufTPVectBus/1 -> Bus Selector1/1
  LM_PathDisBus/1 -> Bus Selector3/1
  MATLAB Function1/3(TpValidNum) -> LM_OTLBufE1TpLastValidNum/1
  MATLAB Function1/4(SPValidPos) -> LM_OTLBufE1SPLastValidPos/1

== system PubIfDecisionLM_MDL/Subsystem2/LM_OTL/LM_OTL_MovObjTrajFit/LM_OTL_BufTPAssess/LM_OTL_BufTrajEva/Subsystem6 ==
  LM_OTLBufValid : Inport
  LM_OTLBufTPVectBus : Inport  Port=2
  ILM_OTLBufTPInfoBus : Inport  Port=3
  LM_PathDisBus : Inport  Port=4
  Bus Selector : BusSelector  OutputSignals=LM_OTLBufE2LastValid
  Bus Selector1 : BusSelector  OutputSignals=LM_OTLBufE2DxVect,LM_OTLBufE2DyVect
  Bus Selector2 : BusSelector  OutputSignals=LM_OTLBufLastSPPosInfo.LM_OTLBufE2LastSPPos,LM_OTLBufLastEPPosInfo.LM_OTLBufE2LastEPPos
  Bus Selector3 : BusSelector  OutputSignals=LM_PathDisBus.LM_FntPath1Dis,LM_PathDisBus.LM_FntPath2Dis,LM_PathDisBus.LM_FntPath3Dis
  Constant : Constant  Value=P_LM_OTLTrajStdThre
  MATLAB Function1 : MATLAB Function  TreatAsAtomicUnit=on
  LM_OTLBufE2LastOffset : Outport
  LM_OTLBufE2LastFlg : Outport  Port=2
  LM_OTLBufE2TpLastValidNum : Outport  Port=3
  LM_OTLBufE2SPLastValidPos : Outport  Port=4
  wires:
  Constant/1 -> MATLAB Function1/9(P_LM_OTLTrajStdThre)
  Bus Selector1/1 -> MATLAB Function1/2(LM_OTLDxVect)  "<LM_OTLBufE2DxVect>"
  Bus Selector/1 -> MATLAB Function1/1(LM_OTLBufValidInfo)  "<LM_OTLBufE2LastValid>"
  MATLAB Function1/2(Flg) -> LM_OTLBufE2LastFlg/1
  Bus Selector3/3 -> MATLAB Function1/8(LM_FntPath3Dis)  "<LM_FntPath3Dis>"
  Bus Selector2/1 -> MATLAB Function1/4(LM_OTLSPPos)  "<LM_OTLBufE2LastSPPos>"
  Bus Selector2/2 -> MATLAB Function1/5(LM_OTLEPPos)  "<LM_OTLBufE2LastEPPos>"
  Bus Selector1/2 -> MATLAB Function1/3(LM_OTLDyVect)  "<LM_OTLBufE2DyVect>"
  LM_OTLBufValid/1 -> Bus Selector/1
  Bus Selector3/2 -> MATLAB Function1/7(LM_FntPath2Dis)  "<LM_FntPath2Dis>"
  Bus Selector3/1 -> MATLAB Function1/6(LM_FntPath1Dis)  "<LM_FntPath1Dis>"
  MATLAB Function1/1(Offset) -> LM_OTLBufE2LastOffset/1
  ILM_OTLBufTPInfoBus/1 -> Bus Selector2/1
  LM_OTLBufTPVectBus/1 -> Bus Selector1/1
  LM_PathDisBus/1 -> Bus Selector3/1
  MATLAB Function1/3(TpValidNum) -> LM_OTLBufE2TpLastValidNum/1
  MATLAB Function1/4(SPValidPos) -> LM_OTLBufE2SPLastValidPos/1

== system PubIfDecisionLM_MDL/Subsystem2/LM_OTL/LM_OTL_MovObjTrajFit/LM_OTL_BufTPAssess/LM_OTL_BufTrajEva/Subsystem7 ==
  LM_OTLBufValid : Inport
  LM_OTLBufTPVectBus : Inport  Port=2
  ILM_OTLBufTPInfoBus : Inport  Port=3
  LM_PathDisBus : Inport  Port=4
  Bus Selector : BusSelector  OutputSignals=LM_OTLBufE2Valid
  Bus Selector1 : BusSelector  OutputSignals=LM_OTLBufE2DxVect,LM_OTLBufE2DyVect
  Bus Selector2 : BusSelector  OutputSignals=LM_OTLBufSPPosInfo.LM_OTLBufE2SPPos,LM_OTLBufEPPosInfo.LM_OTLBufE2EPPos
  Bus Selector3 : BusSelector  OutputSignals=LM_PathDisBus.LM_FntPath1Dis,LM_PathDisBus.LM_FntPath2Dis,LM_PathDisBus.LM_FntPath3Dis
  Constant : Constant  Value=P_LM_OTLTrajStdThre
  MATLAB Function1 : MATLAB Function  TreatAsAtomicUnit=on
  LM_OTLBufE2Offset : Outport
  LM_OTLBufE2Flg : Outport  Port=2
  LM_OTLBufE2TpValidNum : Outport  Port=3
  LM_OTLBufE2SPValidPos : Outport  Port=4
  wires:
  Constant/1 -> MATLAB Function1/9(P_LM_OTLTrajStdThre)
  Bus Selector1/1 -> MATLAB Function1/2(LM_OTLDxVect)  "<LM_OTLBufE2DxVect>"
  Bus Selector/1 -> MATLAB Function1/1(LM_OTLBufValidInfo)  "<LM_OTLBufE2Valid>"
  MATLAB Function1/2(Flg) -> LM_OTLBufE2Flg/1
  Bus Selector3/3 -> MATLAB Function1/8(LM_FntPath3Dis)  "<LM_FntPath3Dis>"
  Bus Selector2/1 -> MATLAB Function1/4(LM_OTLSPPos)  "<LM_OTLBufE2SPPos>"
  Bus Selector2/2 -> MATLAB Function1/5(LM_OTLEPPos)  "<LM_OTLBufE2EPPos>"
  Bus Selector1/2 -> MATLAB Function1/3(LM_OTLDyVect)  "<LM_OTLBufE2DyVect>"
  LM_OTLBufValid/1 -> Bus Selector/1
  Bus Selector3/2 -> MATLAB Function1/7(LM_FntPath2Dis)  "<LM_FntPath2Dis>"
  Bus Selector3/1 -> MATLAB Function1/6(LM_FntPath1Dis)  "<LM_FntPath1Dis>"
  MATLAB Function1/1(Offset) -> LM_OTLBufE2Offset/1
  ILM_OTLBufTPInfoBus/1 -> Bus Selector2/1
  LM_OTLBufTPVectBus/1 -> Bus Selector1/1
  LM_PathDisBus/1 -> Bus Selector3/1
  MATLAB Function1/3(TpValidNum) -> LM_OTLBufE2TpValidNum/1
  MATLAB Function1/4(SPValidPos) -> LM_OTLBufE2SPValidPos/1

== system PubIfDecisionLM_MDL/Subsystem2/LM_OTL/LM_OTL_MovObjTrajFit/LM_OTL_BufTPAssess/LM_OTL_BufTrajEva/Subsystem8 ==
  LM_OTLBufValid : Inport
  LM_OTLBufTPVectBus : Inport  Port=2
  ILM_OTLBufTPInfoBus : Inport  Port=3
  LM_PathDisBus : Inport  Port=4
  Bus Selector : BusSelector  OutputSignals=LM_OTLBufR1LastValid
  Bus Selector1 : BusSelector  OutputSignals=LM_OTLBufR1DxVect,LM_OTLBufR1DyVect
  Bus Selector2 : BusSelector  OutputSignals=LM_OTLBufLastSPPosInfo.LM_OTLBufR1LastSPPos,LM_OTLBufLastEPPosInfo.LM_OTLBufR1LastEPPos
  Bus Selector3 : BusSelector  OutputSignals=LM_PathDisBus.LM_FntPath1Dis,LM_PathDisBus.LM_FntPath2Dis,LM_PathDisBus.LM_FntPath3Dis
  Constant : Constant  Value=P_LM_OTLTrajStdThre
  MATLAB Function1 : MATLAB Function  TreatAsAtomicUnit=on
  LM_OTLBufR1LastOffset : Outport
  LM_OTLBufR1LastFlg : Outport  Port=2
  LM_OTLBufR1TpLastValidNum : Outport  Port=3
  LM_OTLBufR1SPLastValidPos : Outport  Port=4
  wires:
  Constant/1 -> MATLAB Function1/9(P_LM_OTLTrajStdThre)
  Bus Selector1/1 -> MATLAB Function1/2(LM_OTLDxVect)  "<LM_OTLBufR1DxVect>"
  Bus Selector/1 -> MATLAB Function1/1(LM_OTLBufValidInfo)  "<LM_OTLBufR1LastValid>"
  MATLAB Function1/2(Flg) -> LM_OTLBufR1LastFlg/1
  Bus Selector3/3 -> MATLAB Function1/8(LM_FntPath3Dis)  "<LM_FntPath3Dis>"
  Bus Selector2/1 -> MATLAB Function1/4(LM_OTLSPPos)  "<LM_OTLBufR1LastSPPos>"
  Bus Selector2/2 -> MATLAB Function1/5(LM_OTLEPPos)  "<LM_OTLBufR1LastEPPos>"
  Bus Selector1/2 -> MATLAB Function1/3(LM_OTLDyVect)  "<LM_OTLBufR1DyVect>"
  LM_OTLBufValid/1 -> Bus Selector/1
  Bus Selector3/2 -> MATLAB Function1/7(LM_FntPath2Dis)  "<LM_FntPath2Dis>"
  Bus Selector3/1 -> MATLAB Function1/6(LM_FntPath1Dis)  "<LM_FntPath1Dis>"
  MATLAB Function1/1(Offset) -> LM_OTLBufR1LastOffset/1
  ILM_OTLBufTPInfoBus/1 -> Bus Selector2/1
  LM_OTLBufTPVectBus/1 -> Bus Selector1/1
  LM_PathDisBus/1 -> Bus Selector3/1
  MATLAB Function1/3(TpValidNum) -> LM_OTLBufR1TpLastValidNum/1
  MATLAB Function1/4(SPValidPos) -> LM_OTLBufR1SPLastValidPos/1

== system PubIfDecisionLM_MDL/Subsystem2/LM_OTL/LM_OTL_MovObjTrajFit/LM_OTL_BufTPAssess/LM_OTL_BufTrajEva/Subsystem9 ==
  LM_OTLBufValid : Inport
  LM_OTLBufTPVectBus : Inport  Port=2
  ILM_OTLBufTPInfoBus : Inport  Port=3
  LM_PathDisBus : Inport  Port=4
  Bus Selector : BusSelector  OutputSignals=LM_OTLBufR1Valid
  Bus Selector1 : BusSelector  OutputSignals=LM_OTLBufR1DxVect,LM_OTLBufR1DyVect
  Bus Selector2 : BusSelector  OutputSignals=LM_OTLBufSPPosInfo.LM_OTLBufR1SPPos,LM_OTLBufEPPosInfo.LM_OTLBufR1EPPos
  Bus Selector3 : BusSelector  OutputSignals=LM_PathDisBus.LM_FntPath1Dis,LM_PathDisBus.LM_FntPath2Dis,LM_PathDisBus.LM_FntPath3Dis
  Constant : Constant  Value=P_LM_OTLTrajStdThre
  MATLAB Function1 : MATLAB Function  TreatAsAtomicUnit=on
  LM_OTLBufR1Offset : Outport
  LM_OTLBufR1Flg : Outport  Port=2
  LM_OTLBufR1TpValidNum : Outport  Port=3
  LM_OTLBufR1SPValidPos : Outport  Port=4
  wires:
  Constant/1 -> MATLAB Function1/9(P_LM_OTLTrajStdThre)
  Bus Selector1/1 -> MATLAB Function1/2(LM_OTLDxVect)  "<LM_OTLBufR1DxVect>"
  Bus Selector/1 -> MATLAB Function1/1(LM_OTLBufValidInfo)  "<LM_OTLBufR1Valid>"
  MATLAB Function1/2(Flg) -> LM_OTLBufR1Flg/1
  Bus Selector3/3 -> MATLAB Function1/8(LM_FntPath3Dis)  "<LM_FntPath3Dis>"
  Bus Selector2/1 -> MATLAB Function1/4(LM_OTLSPPos)  "<LM_OTLBufR1SPPos>"
  Bus Selector2/2 -> MATLAB Function1/5(LM_OTLEPPos)  "<LM_OTLBufR1EPPos>"
  Bus Selector1/2 -> MATLAB Function1/3(LM_OTLDyVect)  "<LM_OTLBufR1DyVect>"
  LM_OTLBufValid/1 -> Bus Selector/1
  Bus Selector3/2 -> MATLAB Function1/7(LM_FntPath2Dis)  "<LM_FntPath2Dis>"
  Bus Selector3/1 -> MATLAB Function1/6(LM_FntPath1Dis)  "<LM_FntPath1Dis>"
  MATLAB Function1/1(Offset) -> LM_OTLBufR1Offset/1
  ILM_OTLBufTPInfoBus/1 -> Bus Selector2/1
  LM_OTLBufTPVectBus/1 -> Bus Selector1/1
  LM_PathDisBus/1 -> Bus Selector3/1
  MATLAB Function1/3(TpValidNum) -> LM_OTLBufR1TpValidNum/1
  MATLAB Function1/4(SPValidPos) -> LM_OTLBufR1SPValidPos/1

== system PubIfDecisionLM_MDL/Subsystem2/LM_OTL/LM_OTL_MovObjTrajRecord3/LM_OTL_BufTPCC/Subsystem/LM_OTLHostBufCoordinateConvert ==
  note: 0x0: not standstill
  VehStandstill : Inport
  LM_OTLOffsetX : Inport  Port=2
  LM_OTLOffsetY : Inport  Port=3
  LM_OTLOffsetAng : Inport  Port=4
  LM_OTLBufE1DxVectK1 : Inport  Port=5
  LM_OTLBufE1DyVectK1 : Inport  Port=6
  LM_OTLBufE2DxVectK1 : Inport  Port=7
  LM_OTLBufE2DyVectK1 : Inport  Port=8
  If : If  IfExpression=u1 == 0
  If Action Subsystem : Subsystem  TreatAsAtomicUnit=on
  If Action Subsystem1 : Subsystem  TreatAsAtomicUnit=on
  Merge{2..5} (4 alike) : Merge
  LM_OTLBufE1DxVectK1Adju : Outport
  LM_OTLBufE1DyVectK1Adju : Outport  Port=2
  LM_OTLBufE2DxVectK1Adju : Outport  Port=3
  LM_OTLBufE2DyVectK1Adju : Outport  Port=4
  wires:
  If Action Subsystem1/4(LM_OTLBufE2DyVectK1Adju) -> Merge5/2
  If Action Subsystem1/3(LM_OTLBufE2DxVectK1Adju) -> Merge4/2
  If Action Subsystem1/2(LM_OTLBufE1DyVectK1Adju) -> Merge3/2
  If Action Subsystem1/1(LM_OTLBufE1DxVectK1Adju) -> Merge2/2
  LM_OTLBufE2DyVectK1/1 -> If Action Subsystem/7(LM_OTLBufE2DyVectK1), If Action Subsystem1/4(LM_OTLBufE2DyVectK1)
  LM_OTLBufE2DxVectK1/1 -> If Action Subsystem/6(LM_OTLBufE2DxVectK1), If Action Subsystem1/3(LM_OTLBufE2DxVectK1)
  LM_OTLBufE1DyVectK1/1 -> If Action Subsystem/5(LM_OTLBufE1DyVectK1), If Action Subsystem1/2(LM_OTLBufE1DyVectK1)
  LM_OTLBufE1DxVectK1/1 -> If Action Subsystem/4(LM_OTLBufE1DxVectK1), If Action Subsystem1/1(LM_OTLBufE1DxVectK1)
  If Action Subsystem/4(LM_OTLBufE2DyVectK1Adju) -> Merge5/1
  If Action Subsystem/3(LM_OTLBufE2DxVectK1Adju) -> Merge4/1
  Merge4/1 -> LM_OTLBufE2DxVectK1Adju/1
  Merge5/1 -> LM_OTLBufE2DyVectK1Adju/1
  If Action Subsystem/1(LM_OTLBufE1DxVectK1Adju) -> Merge2/1
  If Action Subsystem/2(LM_OTLBufE1DyVectK1Adju) -> Merge3/1
  Merge2/1 -> LM_OTLBufE1DxVectK1Adju/1
  Merge3/1 -> LM_OTLBufE1DyVectK1Adju/1
  LM_OTLOffsetX/1 -> If Action Subsystem/1(LM_OTLOffsetX)
  LM_OTLOffsetY/1 -> If Action Subsystem/2(LM_OTLOffsetY)
  LM_OTLOffsetAng/1 -> If Action Subsystem/3(LM_OTLOffsetAng)
  If/2 -> If Action Subsystem1/Action
  If/1 -> If Action Subsystem/Action
  VehStandstill/1 -> If/1

== system PubIfDecisionLM_MDL/Subsystem2/LM_OTL/LM_OTL_MovObjTrajRecord3/LM_OTL_BufTPCC/Subsystem/LM_OTLLeBufCoordinateConvert ==
  note: 0x0: not standstill
  VehStandstill : Inport
  LM_OTLOffsetX : Inport  Port=2
  LM_OTLOffsetY : Inport  Port=3
  LM_OTLOffsetAng : Inport  Port=4
  LM_OTLBufL1DxVectK1 : Inport  Port=5
  LM_OTLBufL1DyVectK1 : Inport  Port=6
  LM_OTLBufL2DxVectK1 : Inport  Port=7
  LM_OTLBufL2DyVectK1 : Inport  Port=8
  If : If  IfExpression=u1 == 0
  If Action Subsystem : Subsystem  TreatAsAtomicUnit=on
  If Action Subsystem1 : Subsystem  TreatAsAtomicUnit=on
  Merge{2..5} (4 alike) : Merge
  LM_OTLBufL1DxVectK1Adju : Outport
  LM_OTLBufL1DyVectK1Adju : Outport  Port=2
  LM_OTLBufL2DxVectK1Adju : Outport  Port=3
  LM_OTLBufL2DyVectK1Adju : Outport  Port=4
  wires:
  If Action Subsystem1/4(LM_OTLBufL2DyVectK1Adju) -> Merge5/2
  If Action Subsystem1/3(LM_OTLBufL2DxVectK1Adju) -> Merge4/2
  If Action Subsystem1/2(LM_OTLBufL1DyVectK1Adju) -> Merge3/2
  If Action Subsystem1/1(LM_OTLBufL1DxVectK1Adju) -> Merge2/2
  LM_OTLBufL2DyVectK1/1 -> If Action Subsystem/7(LM_OTLBufL2DyVectK1), If Action Subsystem1/4(LM_OTLBufL2DyVectK1)
  LM_OTLBufL2DxVectK1/1 -> If Action Subsystem/6(LM_OTLBufL2DxVectK1), If Action Subsystem1/3(LM_OTLBufL2DxVectK1)
  LM_OTLBufL1DyVectK1/1 -> If Action Subsystem/5(LM_OTLBufL1DyVectK1), If Action Subsystem1/2(LM_OTLBufL1DyVectK1)
  LM_OTLBufL1DxVectK1/1 -> If Action Subsystem/4(LM_OTLBufL1DxVectK1), If Action Subsystem1/1(LM_OTLBufL1DxVectK1)
  If Action Subsystem/4(LM_OTLBufL2DyVectK1Adju) -> Merge5/1
  If Action Subsystem/3(LM_OTLBufL2DxVectK1Adju) -> Merge4/1
  Merge4/1 -> LM_OTLBufL2DxVectK1Adju/1
  Merge5/1 -> LM_OTLBufL2DyVectK1Adju/1
  If Action Subsystem/1(LM_OTLBufL1DxVectK1Adju) -> Merge2/1
  If Action Subsystem/2(LM_OTLBufL1DyVectK1Adju) -> Merge3/1
  Merge2/1 -> LM_OTLBufL1DxVectK1Adju/1
  Merge3/1 -> LM_OTLBufL1DyVectK1Adju/1
  LM_OTLOffsetX/1 -> If Action Subsystem/1(LM_OTLOffsetX)
  LM_OTLOffsetY/1 -> If Action Subsystem/2(LM_OTLOffsetY)
  LM_OTLOffsetAng/1 -> If Action Subsystem/3(LM_OTLOffsetAng)
  If/2 -> If Action Subsystem1/Action
  If/1 -> If Action Subsystem/Action
  VehStandstill/1 -> If/1

== system PubIfDecisionLM_MDL/Subsystem2/LM_OTL/LM_OTL_MovObjTrajRecord3/LM_OTL_BufTPCC/Subsystem/LM_OTLRiBufCoordinateConvert ==
  note: 0x0: not standstill
  VehStandstill : Inport
  LM_OTLOffsetX : Inport  Port=2
  LM_OTLOffsetY : Inport  Port=3
  LM_OTLOffsetAng : Inport  Port=4
  LM_OTLBufR1DxVectK1 : Inport  Port=5
  LM_OTLBufR1DyVectK1 : Inport  Port=6
  LM_OTLBufR2DxVectK1 : Inport  Port=7
  LM_OTLBufR2DyVectK1 : Inport  Port=8
  If : If  IfExpression=u1 == 0
  If Action Subsystem : Subsystem  TreatAsAtomicUnit=on
  If Action Subsystem1 : Subsystem  TreatAsAtomicUnit=on
  Merge{2..5} (4 alike) : Merge
  LM_OTLBufR1DxVectK1Adju : Outport
  LM_OTLBufR1DyVectK1Adju : Outport  Port=2
  LM_OTLBufR2DxVectK1Adju : Outport  Port=3
  LM_OTLBufR2DyVectK1Adju : Outport  Port=4
  wires:
  If Action Subsystem1/4(LM_OTLBufR2DyVectK1Adju) -> Merge5/2
  If Action Subsystem1/3(LM_OTLBufR2DxVectK1Adju) -> Merge4/2
  If Action Subsystem1/2(LM_OTLBufR1DyVectK1Adju) -> Merge3/2
  If Action Subsystem1/1(LM_OTLBufR1DxVectK1Adju) -> Merge2/2
  LM_OTLBufR2DyVectK1/1 -> If Action Subsystem/7(LM_OTLBufR2DyVectK1), If Action Subsystem1/4(LM_OTLBufR2DyVectK1)
  LM_OTLBufR2DxVectK1/1 -> If Action Subsystem/6(LM_OTLBufR2DxVectK1), If Action Subsystem1/3(LM_OTLBufR2DxVectK1)
  LM_OTLBufR1DyVectK1/1 -> If Action Subsystem/5(LM_OTLBufR1DyVectK1), If Action Subsystem1/2(LM_OTLBufR1DyVectK1)
  LM_OTLBufR1DxVectK1/1 -> If Action Subsystem/4(LM_OTLBufR1DxVectK1), If Action Subsystem1/1(LM_OTLBufR1DxVectK1)
  If Action Subsystem/4(LM_OTLBufR2DyVectK1Adju) -> Merge5/1
  If Action Subsystem/3(LM_OTLBufR2DxVectK1Adju) -> Merge4/1
  Merge4/1 -> LM_OTLBufR2DxVectK1Adju/1
  Merge5/1 -> LM_OTLBufR2DyVectK1Adju/1
  If Action Subsystem/1(LM_OTLBufR1DxVectK1Adju) -> Merge2/1
  If Action Subsystem/2(LM_OTLBufR1DyVectK1Adju) -> Merge3/1
  Merge2/1 -> LM_OTLBufR1DxVectK1Adju/1
  Merge3/1 -> LM_OTLBufR1DyVectK1Adju/1
  LM_OTLOffsetX/1 -> If Action Subsystem/1(LM_OTLOffsetX)
  LM_OTLOffsetY/1 -> If Action Subsystem/2(LM_OTLOffsetY)
  LM_OTLOffsetAng/1 -> If Action Subsystem/3(LM_OTLOffsetAng)
  If/2 -> If Action Subsystem1/Action
  If/1 -> If Action Subsystem/Action
  VehStandstill/1 -> If/1
